simulink model "induction_heather_model"  (R2023a)
settings: Solver=FixedStepAuto  StartTime=0.0  StopTime=inf  RelTol=1e-3  EnableMultiTasking=on
libraries: mbedblockslib x7, library x3
settings Model: ExtModeTrigDuration=10  Creator=miria  LastModifiedBy=miria
settings SolverCC: AlgebraicLoopSolver=TrustRegion
settings OptimizationCC: EnhancedBackFolding=on  PassReuseOutputArgsAs=Individual arguments  ZeroExternalMemoryAtStartup=off  ZeroInternalMemoryAtStartup=off  MaxStackSize=64  OptimizeBlockOrder=speed  DifferentSizesBufferReuse=on  OptimizationCustomize=off  EfficientTunableParamExpr=on
settings DebuggingCC: ParameterTunabilityLossMsg=error
settings HardwareCC: ProdBitPerPointer=32  ProdBitPerSizeT=32  ProdBitPerPtrDiffT=32  ProdLargestAtomicInteger=Long  ProdLargestAtomicFloat=Double  ProdWordSize=32  ProdLongLongMode=on  ProdHWDeviceType=ARM Compatible->ARM Cortex  UseEmbeddedCoderFeatures=off
settings SFSimCC: MATLABDynamicMemAlloc=off
settings RTWCC: Description=Embedded Coder  SystemTargetFile=ert.tlc  HardwareBoard=STM32 Nucleo F401RE  TemplateMakefile=ert_default_tmf  Toolchain=GNU Tools for ARM Embedded Processors
settings CodeAppCC: ForceParamTrailComments=on  IgnoreCustomStorageClasses=off  OperatorAnnotations=on  SimulinkDataObjDesc=on  SFDataObjDesc=on  InsertBlockDesc=on
settings ERTTargetCC: SupportNonInlinedSFcns=on  ExtModeTransport=3  ExtModeStaticAlloc=on  ExtModeStaticAllocSize=2000  ExtModeMexFile=ext_xcp  ExtModeIntrfLevel=Level2 - Open

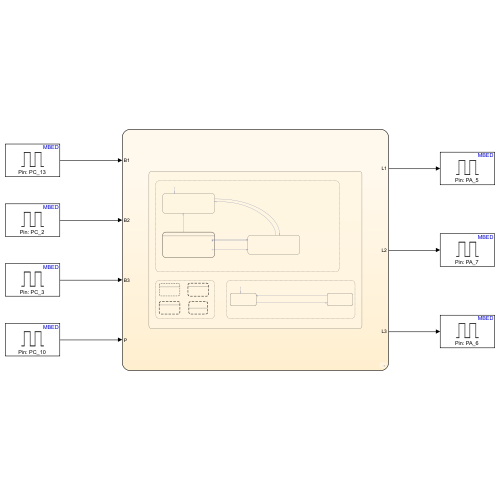
[thumbnail: Simulink's stored preview of the top-level diagram]
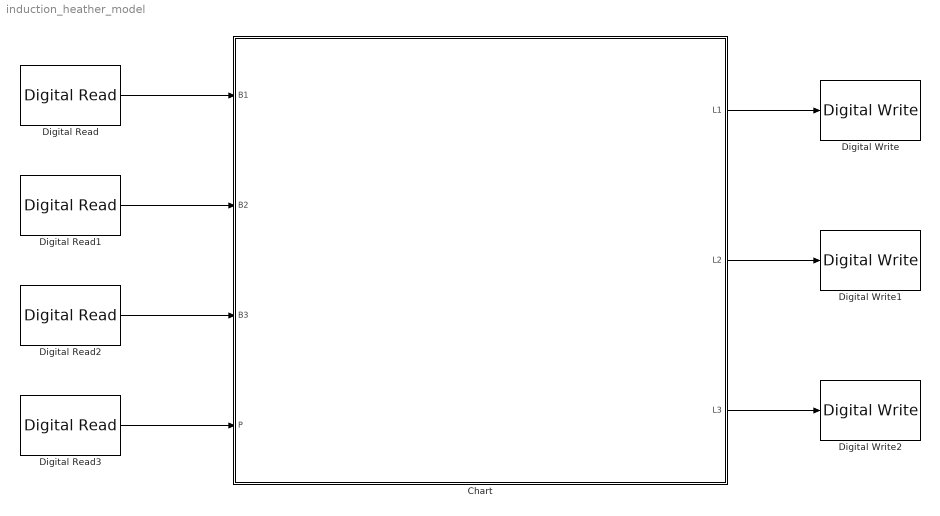
== system induction_heather_model ==
  Chart : Stateflow chart  TreatAsAtomicUnit=on
  Digital Read : mbedblockslib/Digital Read  Pin=PC_13  Direction=input  SampleTime=0.001
      settings: LibrarySourceBlock=stmnucleorootlib/Common/Digital Read
  Digital Read1 : mbedblockslib/Digital Read  Pin=PC_2  Direction=input  SampleTime=0.001
      settings: LibrarySourceBlock=stmnucleorootlib/Common/Digital Read
  Digital Read2 : mbedblockslib/Digital Read  Pin=PC_3  Direction=input  SampleTime=0.001
      settings: LibrarySourceBlock=stmnucleorootlib/Common/Digital Read
  Digital Read3 : mbedblockslib/Digital Read  Pin=PC_10  Direction=input  SampleTime=0.001
      settings: LibrarySourceBlock=stmnucleorootlib/Common/Digital Read
  Digital Write : mbedblockslib/Digital Write  Pin=PA_5  Direction=output
      settings: LibrarySourceBlock=stmnucleorootlib/Common/Digital Write
  Digital Write1 : mbedblockslib/Digital Write  Pin=PA_7  Direction=output
      settings: LibrarySourceBlock=stmnucleorootlib/Common/Digital Write
  Digital Write2 : mbedblockslib/Digital Write  Pin=PA_6  Direction=output
      settings: LibrarySourceBlock=stmnucleorootlib/Common/Digital Write
  wires:
  Digital Read3/1 -> Chart/4(P)
  Chart/1(L1) -> Digital Write/1
  Chart/2(L2) -> Digital Write1/1
  Chart/3(L3) -> Digital Write2/1
  Digital Read/1 -> Chart/1(B1)
  Digital Read1/1 -> Chart/2(B2)
  Digital Read2/1 -> Chart/3(B3)

== stateflow chart induction_heather_model/Chart ==
  state INDUCTION_STOVE
    state HEATER [parallel]
      settings: executionOrder=1
      state OFF
        en: L1 = LED_OFF;
        L2 = LED_OFF;
        l3s = LED_OFF;
        period = 1;
      state COOKING
        state WAITING
          ready = false;
          on after(5, sec):
          ready = true;
        state READY
          en: level = 0;
          next_level = 0;
          l3s = LED_OFF;
          period = 0;
        state POWER
          en: level=next_level;
          l3s = LED_ON;
          period = int32( 2000/2^(level-1));
        state ANOMALY
          en: L2 = LED_ON;
          ex: L2 = LED_OFF;
        WAITING -> WAITING [order 1] : [b2s==PRESSED && next_level < 4]{next_level=next_level+1;}
        WAITING -> WAITING [order 3] : [b3s==PRESSED && next_level > 0]{next_level=next_level-1;}
        READY -> WAITING [order 2] : [b2s==PRESSED]{next_level=next_level+1;}
        WAITING -> READY [order 5] : [ready==true && next_level == 0]
        POWER -> WAITING [order 2] : [b2s==PRESSED && next_level < 4]{next_level=next_level+1;}
        POWER -> WAITING [order 3] : [b3s==PRESSED && next_level  > 0]{next_level=next_level-1;}
        WAITING -> ANOMALY [order 2] : [ps~=PRESENCE]
        WAITING -> POWER [order 4] : [ready==true && next_level ~= 0]
        POWER -> ANOMALY [order 1] : [ps~=PRESENCE]
        ANOMALY -> POWER [order 1] : [ps==PRESENCE]
      state ON
        en: L1 = LED_ON;
        L2 = LED_OFF;
        l3s = LED_OFF;
      (default) -> INDUCTION_STOVE.HEATER.OFF
      INDUCTION_STOVE.HEATER.OFF -> INDUCTION_STOVE.HEATER.ON : [b1s==PRESSED]
      INDUCTION_STOVE.HEATER.ON -> INDUCTION_STOVE.HEATER.OFF [order 2] : [b1s==PRESSED]
      COOKING -> INDUCTION_STOVE.HEATER.OFF : [b1s==PRESSED ]
      ANOMALY -> INDUCTION_STOVE.HEATER.ON [order 2] : [after(10,sec)]
      INDUCTION_STOVE.HEATER.ON -> READY [order 1] : [ps==PRESENCE]
      READY -> INDUCTION_STOVE.HEATER.ON [order 1] : [ps~=PRESENCE ]
    state INPUTS [parallel]
      settings: executionOrder=2
      state BUTTON_3 [parallel]
        settings: executionOrder=4
      state BUTTON_1 [parallel]
        settings: executionOrder=3
        state OFF
          en: b1s = ~PRESSED;
        state WAIT_ON
          en:
          on after(200, msec):
          b1s=PRESSED;
        state LONGPRESSED_OFF
          en: b1s =~PRESSED;
        state LONGPRESSED_ON
          en:
          b1s=~PRESSED;
        state WAIT_OFF
          on after(1,sec):
          b1s=PRESSED;
        state ON
          en: b1s = ~PRESSED;
        (default) -> INDUCTION_STOVE.INPUTS.BUTTON_1.OFF
        INDUCTION_STOVE.INPUTS.BUTTON_1.OFF -> WAIT_ON : [B1==PRESSED]
        WAIT_ON -> INDUCTION_STOVE.INPUTS.BUTTON_1.OFF [order 2] : [B1 ~= PRESSED]
        LONGPRESSED_OFF -> INDUCTION_STOVE.INPUTS.BUTTON_1.OFF : [B1~= PRESSED]
        WAIT_ON -> LONGPRESSED_ON [order 1] : [B1 == PRESSED && b1s == PRESSED]
        WAIT_OFF -> LONGPRESSED_OFF [order 1] : [B1==PRESSED && b1s == PRESSED]
        LONGPRESSED_ON -> INDUCTION_STOVE.INPUTS.BUTTON_1.ON : [B1 ~= PRESSED]
        INDUCTION_STOVE.INPUTS.BUTTON_1.ON -> WAIT_OFF : [B1==PRESSED]
        WAIT_OFF -> INDUCTION_STOVE.INPUTS.BUTTON_1.ON [order 2] : [B1 ~= PRESSED]
      state BUTTON_2 [parallel]
        settings: executionOrder=1
      state PRESENCE [parallel]
        settings: executionOrder=2
    state POWER_LED [parallel]
      settings: executionOrder=3
      state OFF
        entry: L3 = LED_OFF;
      state ON
        entry: L3 = LED_ON;
      (default) -> INDUCTION_STOVE.POWER_LED.OFF
      INDUCTION_STOVE.POWER_LED.ON -> INDUCTION_STOVE.POWER_LED.OFF : [l3s == LED_OFF || (after(period/2,msec) && l3s == LED_ON)]
      INDUCTION_STOVE.POWER_LED.OFF -> INDUCTION_STOVE.POWER_LED.ON : [after(period/2,msec) && l3s == LED_ON]
  data: button_state function_output; button_state function_output; presence_state function_output; B1 input boolean size=1; B2 input boolean size=1; B3 input boolean size=1; P input boolean size=1; L1 output boolean size=1; L2 output boolean size=1; L3 output boolean size=1; LED_ON constant boolean =1; LED_OFF constant boolean =0; PRESSED constant boolean =0; b1s local boolean size=1; ps local boolean size=1; PRESENCE constant boolean =0; b3s local boolean size=1; b2s local boolean size=1; l3s local boolean size=1; period local int32 size=1; level local; next_level local; ready local boolean
